simulink model "Schimmel_Evan_lab_2_model"  (R2021a)
settings: Solver=ode15s  StartTime=0.0  StopTime=tf  MaxStep=maxstep  RelTol=tol  AbsTol=tol
values from neighbouring files (symbols this model uses):
  c = cLab*2.65    [Schimmel_Evan_lab_2_script.m]
  Fin = 8    [Schimmel_Evan_lab_2_script.m]
  g = 9.81    [Schimmel_Evan_lab_2_script.m]
  k = kLab    [Schimmel_Evan_lab_2_script.m]
  m = mLab    [Schimmel_Evan_lab_2_script.m]
  mu = 0.15    [Schimmel_Evan_lab_2_script.m]
  v0 = 0    [Schimmel_Evan_lab_2_script.m]
  x0 = 0    [Schimmel_Evan_lab_2_script.m]
libraries: simulink x1
settings Model: Creator=schimmer  LastModifiedBy=schimmer
settings SolverCC: ZeroCrossAlgorithm=Adaptive  AlgebraicLoopSolver=TrustRegion
settings DataIOCC: SaveOutput=off  SignalLogging=off  DSMLogging=off  SaveTime=off  ReturnWorkspaceOutputs=off  OutputOption=SpecifiedOutputTimes  OutputTimes=tdata
settings DebuggingCC: SFMachineParentedDataDiag=warning

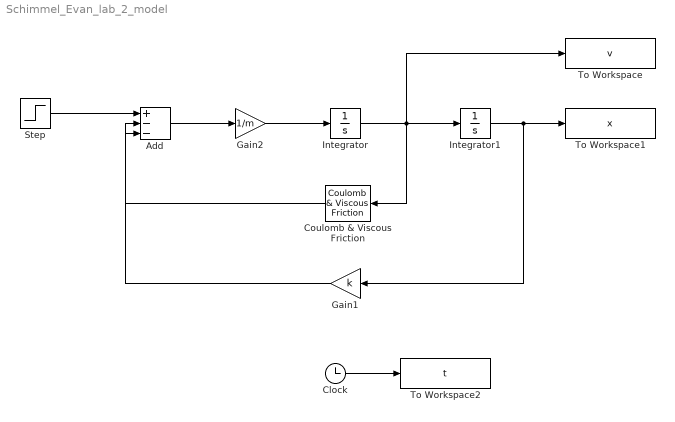
== system Schimmel_Evan_lab_2_model ==
  Add : Sum  Inputs=+--
  Clock : Clock
  Coulomb & Viscous Friction : simulink/Discontinuities/Coulomb & Viscous Friction  offset=mu*m*g  gain=c
  Gain1 : Gain  Gain=k
  Gain2 : Gain  Gain=1/m
  Integrator : Integrator  InitialCondition=v0
  Integrator1 : Integrator  InitialCondition=x0
  Step : Step  Time=0  After=Fin  SampleTime=0
  To Workspace : ToWorkspace  VariableName=v  SampleTime=-1
  To Workspace1 : ToWorkspace  VariableName=x  SampleTime=-1
  To Workspace2 : ToWorkspace  VariableName=t  SampleTime=-1
  wires:
  Integrator/1 -> Coulomb & Viscous Friction/1, Integrator1/1, To Workspace/1
  Integrator1/1 -> Gain1/1, To Workspace1/1
  Add/1 -> Gain2/1
  Gain2/1 -> Integrator/1
  Gain1/1 -> Add/2
  Coulomb & Viscous Friction/1 -> Add/3
  Step/1 -> Add/1
  Clock/1 -> To Workspace2/1
